simulink model "APA_AEB_Version_0_1"  (R2019a)
settings: Solver=FixedStepAuto  StartTime=0.0  StopTime=2  FixedStep=0.01  RelTol=1e-3
libraries: simulink x4, dspnetwork x1, autolibshared x1
(part 3 of 3)

== matlab function APA_AEB_Version_0_1/Resettable Single USS Tracking System/Single USS Tracking System ==
  settings: updateMethod=DISCRETE
  data: Obj_Single_USS_Lgtl input single; Track_Sigle_USS output single; Obj_Single_USS_Latl input single; Vehicle_Lgtl_Vel input single; Vehicle_Latl_Vel input single; Predict_time input single; State_Trans_F input single; State_Trans_P input single; Observation_H input single; DetectNoise_R input single; ProcessNoise_Q input single
function Track_Sigle_USS = Single_USS_Tracking_System(Obj_Single_USS_Lgtl,Obj_Single_USS_Latl,Vehicle_Lgtl_Vel,Vehicle_Latl_Vel,Predict_time,State_Trans_F,State_Trans_P,Observation_H,DetectNoise_R,ProcessNoise_Q)

Delta_x = Vehicle_Lgtl_Vel * Predict_time;
Delta_y = Vehicle_Latl_Vel * Predict_time;
Detection = zeros(12,4);
State_Trans_P_Update = zeros(4,4);
Track_Sigle_USS = single(zeros(12,4));
persistent Track_Object

if isempty(Track_Object)
    Track_Object = zeros(12,4);
    for index = 1:12
        [datalgtl,Lgtl_position_index] = min(abs(Obj_Single_USS_Lgtl(:,index)));
        [datalatl,Latl_position_index] = min(abs(Obj_Single_USS_Latl(:,index)));
        if datalgtl~=0 && datalatl~=0
            %
            Track_Object(index,1) = Obj_Single_USS_Lgtl(Lgtl_position_index,index);
            Track_Object(index,2) = Obj_Single_USS_Latl(Latl_position_index,index);
            Track_Object(index,3) = -1*Vehicle_Lgtl_Vel;
            Track_Object(index,4) = -1*Vehicle_Latl_Vel;
        else
            Track_Object(index,1) = Obj_Single_USS_Lgtl(Lgtl_position_index,index);
            Track_Object(index,2) = Obj_Single_USS_Latl(Latl_position_index,index);
            Track_Object(index,3) = 0;
            Track_Object(index,4) = 0;
        end
    end
    return
end

for Track_id = 1:12
    
    [datalgtl,Lgtl_position_index] = min(abs(Obj_Single_USS_Lgtl(:,Track_id)));
    [datalatl,Latl_position_index] = min(abs(Obj_Single_USS_Latl(:,Track_id)));
    
    if datalgtl~=0 && datalatl~=0
        %
        Detection(Track_id,1) = Obj_Single_USS_Lgtl(Lgtl_position_index,Track_id);
        Detection(Track_id,2) = Obj_Single_USS_Latl(Latl_position_index,Track_id);
        Detection(Track_id,3) = -1*Vehicle_Lgtl_Vel;
        Detection(Track_id,4) = -1*Vehicle_Latl_Vel;
    else
        Detection(Track_id,1) = Obj_Single_USS_Lgtl(Lgtl_position_index,Track_id);
        Detection(Track_id,2) = Obj_Single_USS_Latl(Latl_position_index,Track_id);
        Detection(Track_id,3) = 0;
        Detection(Track_id,4) = 0;
    end
    
    Track_Object_state = (Track_Object(Track_id,:))';
    Track_Object_state_Pred = State_Trans_F * Track_Object_state;
    State_Trans_P = State_Trans_F*State_Trans_P*State_Trans_F'+ProcessNoise_Q;
    Detection_t = Detection(Track_id,:);
    M_dist = sqrt((Track_Object_state_Pred(1,1)-Detection_t(1,1))^2 + (Track_Object_state_Pred(2,1)-Detection_t(1,2))^2);
    if M_dist < 2000
        %       
        Detection_pred = Observation_H*Track_Object_state_Pred;
        Innovation_S = Observation_H*State_Trans_P*Observation_H'+DetectNoise_R;
        KalmanGain_K = State_Trans_P*Observation_H'/Innovation_S;
        Track_Object_state_Update = Track_Object_state_Pred+KalmanGain_K*(Detection(Track_id,:)'-Detection_pred);
        State_Trans_P_Update = (eye(4,4)-KalmanGain_K*Observation_H)*State_Trans_P;
        Track_Object(Track_id,:) = Track_Object_state_Update;
    else
        Track_Object(Track_id,:) = Track_Object(Track_id,:);
    end
end
Track_Sigle_USS = single(Track_Object);
end

== matlab function APA_AEB_Version_0_1/Vehicle_Movement_Calculation ==
  data: Longitual_Velocity input single; Vehicle_Corner output single; Lateral_Velocity input single; Vehicle_predict_time input single; Brake_dist input single; Wheel_Angle input single; Axle_Length input single; Wheel_Base input single; Frt_Bump_dist input single; Rear_Bump_dist input single; Side_wheel_dist input single; CG_Offset_dist input single; Vehicle_Corner_t output single
function [Vehicle_Corner,Vehicle_Corner_t] = Vehicle_Movement_Calculation(Longitual_Velocity,Lateral_Velocity,Vehicle_predict_time,Brake_dist,Wheel_Angle,...
    Axle_Length,Wheel_Base,Frt_Bump_dist,Rear_Bump_dist,Side_wheel_dist,CG_Offset_dist)

Vehicle_Movement_Longitual = Longitual_Velocity*Vehicle_predict_time;
Vehicle_Movement_Lateral = Lateral_Velocity*Vehicle_predict_time;
Vehivle_Lgtl_Brake_dist = Brake_dist;
Vehivle_Latl_Brake_dist = Brake_dist*sin(Wheel_Angle);

Vehicle_Movement_Longitual = Vehicle_Movement_Longitual + Vehivle_Lgtl_Brake_dist;
Vehicle_Movement_Lateral = Vehicle_Movement_Lateral + Vehivle_Latl_Brake_dist;

Corner_LR_X = -1*Rear_Bump_dist;
Corner_LR_Y = -0.5*Wheel_Base;
Corner_RR_X = Corner_LR_X;
Corner_RR_Y = 0.5*Wheel_Base;
Corner_LF_X = Axle_Length + Frt_Bump_dist;
Corner_LF_Y = -0.5*Wheel_Base;
Corner_RF_X = Axle_Length + Frt_Bump_dist;
Corner_RF_Y = 0.5*Wheel_Base;

Corner_LR_X_t = -1*Rear_Bump_dist + Vehicle_Movement_Longitual;
Corner_LR_Y_t = -0.5*Wheel_Base + Vehicle_Movement_Lateral;
Corner_RR_X_t = Corner_LR_X + Vehicle_Movement_Longitual;
Corner_RR_Y_t = 0.5*Wheel_Base + Vehicle_Movement_Lateral;
Corner_LF_X_t = Axle_Length + Frt_Bump_dist + Vehicle_Movement_Longitual;
Corner_LF_Y_t = -0.5*Wheel_Base + Vehicle_Movement_Lateral;
Corner_RF_X_t = Axle_Length + Frt_Bump_dist + Vehicle_Movement_Longitual;
Corner_RF_Y_t = 0.5*Wheel_Base + Vehicle_Movement_Lateral;


Vehicle_Corner_Lgtl = [Corner_LR_X Corner_RR_X Corner_LF_X Corner_RF_X];
Vehicle_Corner_Latl = [Corner_LR_Y Corner_RR_Y Corner_LF_Y Corner_RF_Y];
Vehicle_Corner_Lgtl_t = [Corner_LR_X_t Corner_RR_X_t Corner_LF_X_t Corner_RF_X_t];
Vehicle_Corner_Latl_t = [Corner_LR_Y_t Corner_RR_Y_t Corner_LF_Y_t Corner_RF_Y_t];

Vehicle_Corner = [Vehicle_Corner_Lgtl;Vehicle_Corner_Latl];
Vehicle_Corner_t = [Vehicle_Corner_Lgtl_t;Vehicle_Corner_Latl_t];

== matlab function APA_AEB_Version_0_1/Collision Assessment/Switch Case Action Subsystem/Single_USS_Collision_Assessment ==
  data: Vehicle_Corner input single; Brake_Req_Flag output single; Vehicle_Corner_t input single; Obj_Single_USS_Lgtl input single; Obj_Single_USS_Latl input single

function Brake_Req_Flag = Single_USS_Collision_Assessment(Vehicle_Corner,Vehicle_Corner_t,Obj_Single_USS_Lgtl,Obj_Single_USS_Latl)
% coder.extrinsic('convhull')
%将输入的车辆坐标拆分
Vehicle_Corner_Lgtl = Vehicle_Corner ( 1 , : )'*100 ;
Vehicle_Corner_Latl = Vehicle_Corner ( 2 , : )' *100;
Vehicle_Corner_Lgtl_t = Vehicle_Corner_t( 1 , : )'*100 ;
Vehicle_Corner_Latl_t = Vehicle_Corner_t( 2 , : )'*100 ;
x_outline=[Vehicle_Corner_Lgtl ; Vehicle_Corner_Lgtl_t];
y_outline = [ Vehicle_Corner_Latl ; Vehicle_Corner_Latl_t ];

x_Obj_Single_USS = zeros(60,1);
y_Obj_Single_USS = zeros(60,1);
for k=1:1:12
    for i=1:1:5
    x_Obj_Single_USS((k-1)*5+i) = Obj_Single_USS_Lgtl(i,k);
    y_Obj_Single_USS((k-1)*5+i) = Obj_Single_USS_Latl(i,k);
    end
end
for i=1:1:60
    if x_Obj_Single_USS(i)==0&&y_Obj_Single_USS(i)==0
        x_Obj_Single_USS(i) = +inf ;
        y_Obj_Single_USS(i) = +inf ; 
    end
end
% %判断目标位置是否在车辆轮轮廓以内
[obstacle_in_trajector ] = inpolygon( x_Obj_Single_USS'*0.1 , y_Obj_Single_USS'*0.1 , x_outline , y_outline );
% [obstacle_in_trajector ] = inpolygon( Obj_Single_USS_Lgtl.*0.1 , Obj_Single_USS_Latl.*0.1 , x_outline' , y_outline' );
%是否刹车，若有目标点在轮廓内则发0刹车，反之发1不刹
if sum( obstacle_in_trajector )>0
Brake_Req_Flag = single(0);
else
Brake_Req_Flag = single(1);
end
% function Brake_Req_Flag = Single_USS_Collision_Assessment(Vehicle_Corner,Vehicle_Corner_t,Obj_Single_USS_Lgtl,Obj_Single_USS_Latl)
% %将输入的车辆坐标拆分
% Vehicle_Corner_Lgtl = Vehicle_Corner ( 1 , : )' ;
% Vehicle_Corner_Latl = Vehicle_Corner ( 2 , : )' ;
% Vehicle_Corner_Lgtl_t = Vehicle_Corner_t( 1 , : )' ;
% Vehicle_Corner_Latl_t = Vehicle_Corner_t( 1 , : )' ;
% %找到预测后车辆角点在这一时刻车辆位姿内的角点
% [Vehicle_Corner_t_in_Vehicle_Corner ] = inpolygon( Vehicle_Corner_Lgtl_t , Vehicle_Corner_Latl_t , Vehicle_Corner_Lgtl , Vehicle_Corner_Latl );
% Vehicle_Corner_t_out_Vehicle_Corner_index = find( ~Vehicle_Corner_t_in_Vehicle_Corner );
% %找到这一时刻车辆角点在预测后车辆位姿内的角点在
% [Vehicle_Corner_in_Vehicle_Corner_t ] = inpolygon( Vehicle_Corner_Lgtl , Vehicle_Corner_Latl  , Vehicle_Corner_Lgtl_t , Vehicle_Corner_Latl_t );
% Vehicle_Corner_out_Vehicle_Corner_t_index = find( ~Vehicle_Corner_in_Vehicle_Corner_t );
% %写这一时刻和预测后车辆位姿的外轮廓矩阵
% Vehicle_Corner_t_out_num = length(Vehicle_Corner_t_out_Vehicle_Corner_index) ; 
% Vehicle_Corner_out_num =  length(Vehicle_Corner_out_Vehicle_Corner_t_index)   ; 
% outline_num = Vehicle_Corner_t_out_num + Vehicle_Corner_out_num ;                %轮廓的总点数
% x_outline = zeros(1,outline_num) ; 
% y_outline = zeros(1,outline_num) ; 
% for i=1:1:outline_num 
%     if i<= Vehicle_Corner_t_out_num
%     x_outline(i) = Vehicle_Corner_Lgtl_t( Vehicle_Corner_t_out_Vehicle_Corner_index(i) ) ; 
%     y_outline(i) = Vehicle_Corner_Latl_t( Vehicle_Corner_t_out_Vehicle_Corner_index(i) ) ;
%     else
%     x_outline(i) = Vehicle_Corner_Lgtl( Vehicle_Corner_out_Vehicle_Corner_t_index(i-Vehicle_Corner_t_out_num) ) ; 
%     y_outline(i) = Vehicle_Corner_Latl( Vehicle_Corner_out_Vehicle_Corner_t_index(i-Vehicle_Corner_t_out_num) ) ;
%     end
% end
% %判断目标位置是否在车辆轮轮廓以内
% [obstacle_in_trajector ] = inpolygon( Obj_Single_USS_Lgtl , Obj_Single_USS_Latl , x_outline' , y_outline' );
% %是否刹车，若有目标点在轮廓内则发0刹车，反之发1不刹
% if sum( obstacle_in_trajector )>0
% Brake_Req_Flag = 0;
% else
% Brake_Req_Flag = 1;
% end

== matlab function APA_AEB_Version_0_1/Collision Assessment/Switch Case Action Subsystem1/Multi_USS_Collision_Assessment ==
  data: Vehicle_Corner input single; Brake_Req_Flag output single; Vehicle_Corner_t input single; Obj_Triangle_USS_Lgtl input single; Obj_Triangle_USS_Latl input single

function Brake_Req_Flag = Multi_USS_Collision_Assessment(Vehicle_Corner,Vehicle_Corner_t,Obj_Triangle_USS_Lgtl,Obj_Triangle_USS_Latl)
% coder.extrinsic('convhull')
Vehicle_Corner_Lgtl = Vehicle_Corner ( 1 , : )'*100 ;
Vehicle_Corner_Latl = Vehicle_Corner ( 2 , : )' *100;
Vehicle_Corner_Lgtl_t = Vehicle_Corner_t( 1 , : )'*100 ;
Vehicle_Corner_Latl_t = Vehicle_Corner_t( 2 , : )'*100 ;
x_outline=[Vehicle_Corner_Lgtl ;Vehicle_Corner_Lgtl_t];
y_outline = [ Vehicle_Corner_Latl;Vehicle_Corner_Latl_t ];

%将0变为正无穷
for i=1:1:6
    if Obj_Triangle_USS_Lgtl(i)==0&&Obj_Triangle_USS_Latl(i)==0
        Obj_Triangle_USS_Lgtl(i) = +inf ;
        Obj_Triangle_USS_Latl(i) = +inf ; 
    end
end
%判断目标位置是否在车辆轮轮廓以内
[obstacle_in_trajector ] = inpolygon( Obj_Triangle_USS_Lgtl'*0.1 , Obj_Triangle_USS_Latl'*0.1 , x_outline , y_outline );
%是否刹车，若有目标点在轮廓内则发0刹车，反之发1不刹
if sum( obstacle_in_trajector )>0
Brake_Req_Flag = single(0);
else
Brake_Req_Flag = single(1);
end

== matlab function APA_AEB_Version_0_1/Ultarsonic Processment /Subsystem1/Subsystem1/Detection Processment/Switch Case Action Subsystem1/MATLAB Function ==
  data: Sensor_Detection input; Longitudial_triDist output; Lateral_triDist output
function [Longitudial_triDist,Lateral_triDist] = fcn(Sensor_Detection)
    %
    Longitudial_triDist = single(zeros(1,6));
    %
    Lateral_triDist = single(zeros(1,6));
    %
    Front_leftFront_uss_position_x  = single(3528.8);
    %
    Front_leftFront_uss_position_y  = single(-650.5);
    %
    Front_leftMiddle_uss_position_x  = single(3673.9);
    %
    Front_leftMiddle_uss_position_y  = single(-320.3);
    %
    Front_rightMiddle_uss_position_x  = single(3673.9);
    %
    Front_rightMiddle_uss_position_y  = single(320.3);
    %
    Front_rightFront_uss_position_x  =  single(3528.7);
    %
    Front_rightFront_uss_position_y  =  single(650.4);
    %
    Rear_leftRear_uss_position_x  =  single(-784.2);
    %
    Rear_leftRear_uss_position_y  =  single(-660.4);
    %
    Rear_leftMiddle_uss_position_x  =  single(-904.5);
    %
    Rear_leftMiddle_uss_position_y  =  single(-280.4);
    %
    Rear_rightMiddle_uss_position_x  =  single(-904.5);
    %
    Rear_rightMiddle_uss_position_y  =  single(280.4);
    %
    Rear_rightRear_uss_position_x  =  single(-784.2);
    %
    Rear_rightRear_uss_position_y  =  single(660.4);
    %
    USS_dist  = [single(sqrt((Front_leftFront_uss_position_x-Front_leftMiddle_uss_position_x)^2+(Front_leftFront_uss_position_y-Front_leftMiddle_uss_position_y)^2)),...
        single(sqrt((Front_rightMiddle_uss_position_x-Front_leftMiddle_uss_position_x)^2+(Front_rightMiddle_uss_position_y-Front_leftMiddle_uss_position_y)^2)),...
        single(sqrt((Front_rightMiddle_uss_position_x-Front_rightFront_uss_position_x)^2+(Front_rightMiddle_uss_position_y-Front_rightFront_uss_position_x)^2)),...
        single(sqrt((Rear_rightMiddle_uss_position_x-Rear_rightRear_uss_position_x)^2+(Rear_rightMiddle_uss_position_y-Rear_rightRear_uss_position_y)^2)),...
        single(sqrt((Rear_rightMiddle_uss_position_x-Rear_leftMiddle_uss_position_x)^2+(Rear_rightMiddle_uss_position_y-Rear_leftMiddle_uss_position_y)^2)),...
        single(sqrt((Rear_leftRear_uss_position_x-Rear_leftMiddle_uss_position_x)^2+(Rear_leftRear_uss_position_y-Rear_leftMiddle_uss_position_y)^2))];

    
    
    if Sensor_Detection(2)>0 && Sensor_Detection(3)>0 && Sensor_Detection(4)==0 && Sensor_Detection(2)+Sensor_Detection(3) > USS_dist(1)
        alpha = single(acos((USS_dist(1)^2+Sensor_Detection(2)^2-Sensor_Detection(3)^2)/(2 * USS_dist(1) * Sensor_Detection(2))));
        x = single(sin(alpha)*Sensor_Detection(2));
        y = single(cos(alpha)*Sensor_Detection(2)); 
        a = (Front_leftMiddle_uss_position_x - Front_leftFront_uss_position_x)/USS_dist(1);
        b= abs(Front_leftMiddle_uss_position_y - Front_leftFront_uss_position_y)/USS_dist(1);
        Longitudial_triDist(1) = x * b + y * a + Front_leftFront_uss_position_x;
        Lateral_triDist(1) = - x * a + y * b + Front_leftFront_uss_position_y;
    end
    
    if Sensor_Detection(3)>0 && Sensor_Detection(4)>0 && Sensor_Detection(2)==0 && Sensor_Detection(5)==0 && Sensor_Detection(3)+Sensor_Detection(4) > USS_dist(2)
            alpha = acos((USS_dist(2)^2+Sensor_Detection(3)^2-Sensor_Detection(4)^2)/(2 * USS_dist(2) * Sensor_Detection(3)));
            x = sin(alpha)*Sensor_Detection(3);
            y = cos(alpha)*Sensor_Detection(3);
            a = (Front_rightMiddle_uss_position_x - Front_leftMiddle_uss_position_x)/USS_dist(2);
            b = abs(Front_rightMiddle_uss_position_y - Front_leftMiddle_uss_position_y)/USS_dist(2);
            Longitudial_triDist(2) = x * b + y * a + Front_leftMiddle_uss_position_x;
            Lateral_triDist(2) = - x * a + y * b + Front_leftMiddle_uss_position_y;
    end
    
    if Sensor_Detection(4)>0 && Sensor_Detection(5)>0 && Sensor_Detection(3)==0 && Sensor_Detection(4)+Sensor_Detection(5) > USS_dist(3)
        alpha = acos((USS_dist(3)^2+Sensor_Detection(4)^2-Sensor_Detection(5)^2)/(2 * USS_dist(3) * Sensor_Detection(4)));
        x = sin(alpha)*Sensor_Detection(4);
        y = cos(alpha)*Sensor_Detection(4);
        a = (Front_rightFront_uss_position_x - Front_rightMiddle_uss_position_x)/USS_dist(3);
        b = abs(Front_rightFront_uss_position_y - Front_rightMiddle_uss_position_y)/USS_dist(3);
        Longitudial_triDist(3) = x * b + y * a + Front_rightMiddle_uss_position_x;
        Lateral_triDist(3) = - x * a + y * b + Front_rightMiddle_uss_position_y;
    end
    
    if Sensor_Detection(8)>0 && Sensor_Detection(9)>0 && Sensor_Detection(10)==0 && Sensor_Detection(8)+Sensor_Detection(9) > USS_dist(4)
        alpha = acos((USS_dist(4)^2+Sensor_Detection(8)^2-Sensor_Detection(9)^2)/(2 * USS_dist(4) * Sensor_Detection(8)));
        x = sin(alpha) * Sensor_Detection(8);
        y = cos(alpha )* Sensor_Detection(8); 
        a = -(Rear_rightMiddle_uss_position_x - Rear_rightRear_uss_position_x)/USS_dist(4);
        b= abs(Rear_rightMiddle_uss_position_y - Rear_rightRear_uss_position_y)/USS_dist(4);
        Longitudial_triDist(4) = - ( x * b + y * a ) + Rear_rightRear_uss_position_x;
        Lateral_triDist(4) = - ( - x * a + y * b ) + Rear_rightRear_uss_position_y;
    end
    
    if Sensor_Detection(9)>0 && Sensor_Detection(10)>0 && Sensor_Detection(8)==0 && Sensor_Detection(11)==0 && Sensor_Detection(9)+Sensor_Detection(10) > USS_dist(5)
        alpha = acos((USS_dist(5)^2+Sensor_Detection(9)^2-Sensor_Detection(10)^2)/(2 * USS_dist(5) * Sensor_Detection(9)));
        x = sin(alpha)*Sensor_Detection(9);
        y = cos(alpha)*Sensor_Detection(9); 
        a = -(Rear_leftMiddle_uss_position_x - Rear_rightMiddle_uss_position_x)/USS_dist(5);
        b= abs(Rear_leftMiddle_uss_position_y - Rear_rightMiddle_uss_position_y)/USS_dist(5);
        Longitudial_triDist(5) = - ( x * b + y * a ) + Rear_rightMiddle_uss_position_x;
        Lateral_triDist(5) = - ( x * a + y * b ) + Rear_rightMiddle_uss_position_y;
    end
    
    if Sensor_Detection(10)>0 && Sensor_Detection(11)>0 && Sensor_Detection(9)==0 && Sensor_Detection(10)+Sensor_Detection(11) > USS_dist(6)
        alpha = acos((USS_dist(6)^2+Sensor_Detection(10)^2-Sensor_Detection(11)^2)/(2 * USS_dist(6) * Sensor_Detection(10)));
        x = sin(alpha)*Sensor_Detection(10);
        y = cos(alpha)*Sensor_Detection(10); 
        a = -(Rear_leftRear_uss_position_x - Rear_leftMiddle_uss_position_x)/USS_dist(6);
        b= abs(Rear_leftRear_uss_position_y - Rear_leftMiddle_uss_position_y)/USS_dist(6);
        Longitudial_triDist(6) = - ( x * b + y * a ) + Rear_leftMiddle_uss_position_x;
        Lateral_triDist(6) = - ( - x * a + y * b ) + Rear_leftMiddle_uss_position_y;
    end

== matlab function APA_AEB_Version_0_1/Multi_USS_Tracking_System/Multi USS Tracking ==
  settings: updateMethod=DISCRETE
  data: Obj_Triangle_USS_Lgtl input single; Track_Multi_USS output single; Obj_Triangle_USS_Latl input single; Vehicle_Lgtl_Vel input single; Vehicle_Latl_Vel input single; Predict_time input single; State_Trans_F input single; State_Trans_P input single; Observation_H input single; DetectNoise_R input single; ProcessNoise_Q input single
function Track_Multi_USS = Multi_USS_Tracking_System(Obj_Triangle_USS_Lgtl,Obj_Triangle_USS_Latl,Vehicle_Lgtl_Vel,Vehicle_Latl_Vel,Predict_time,State_Trans_F,State_Trans_P,Observation_H,DetectNoise_R,ProcessNoise_Q)

Delta_x_M = Vehicle_Lgtl_Vel * Predict_time;
Delta_y_M = Vehicle_Latl_Vel * Predict_time;
Detection_M = zeros(6,4);
State_Trans_P_Update_M = zeros(4,4);
Track_Multi_USS = single(zeros(6,4));

persistent Track_Object_Multi

if isempty(Track_Object_Multi)
    % Init the global params for tracker
    Track_Object_Multi = zeros(6,4);
    
    for index_M = 1:6
        if Obj_Triangle_USS_Lgtl(index_M)~=0 && Obj_Triangle_USS_Latl(index_M)~=0
            %
            Track_Object_Multi(index_M,1) = Obj_Triangle_USS_Lgtl(index_M);
            Track_Object_Multi(index_M,2) = Obj_Triangle_USS_Latl(index_M);
            Track_Object_Multi(index_M,3) = -1*Vehicle_Lgtl_Vel;
            Track_Object_Multi(index_M,4) = -1*Vehicle_Latl_Vel;
        else
            Track_Object_Multi(index_M,1) = Obj_Triangle_USS_Lgtl(index_M);
            Track_Object_Multi(index_M,2) = Obj_Triangle_USS_Latl(index_M);
            Track_Object_Multi(index_M,3) = 0;
            Track_Object_Multi(index_M,4) = 0;
        end
    end
    return;
end

for Track_id_M = 1:6
    %
    if Obj_Triangle_USS_Lgtl(Track_id_M)~=0 && Obj_Triangle_USS_Latl(Track_id_M)~=0
        Detection_M(Track_id_M,1) = Obj_Triangle_USS_Lgtl(Track_id_M);
        Detection_M(Track_id_M,2) = Obj_Triangle_USS_Latl(Track_id_M);
        Detection_M(Track_id_M,3) = -1*Vehicle_Lgtl_Vel;
        Detection_M(Track_id_M,4) = -1*Vehicle_Latl_Vel;
    else
        Detection_M(Track_id_M,1) = Obj_Triangle_USS_Lgtl(Track_id_M);
        Detection_M(Track_id_M,2) = Obj_Triangle_USS_Latl(Track_id_M);
        Detection_M(Track_id_M,3) = 0;
        Detection_M(Track_id_M,4) = 0;
    end
    %Kalman——Filter
    Track_Object_state_M = (Track_Object_Multi(Track_id_M,:))';
    Track_Object_state_Pred_M = State_Trans_F * Track_Object_state_M;
    State_Trans_P = State_Trans_F*State_Trans_P*State_Trans_F'+ProcessNoise_Q;
    Detection_M_t = Detection_M(Track_id_M,:);
    MM_dist = sqrt((Track_Object_state_Pred_M(1,1)-Detection_M_t(1,1))^2 + (Track_Object_state_Pred_M(2,1)-Detection_M_t(1,2))^2);
    if MM_dist < 50000
        %
        Detection_pred_M = Observation_H*Track_Object_state_Pred_M;
        Innovation_S = Observation_H*State_Trans_P*Observation_H'+DetectNoise_R;
        KalmanGain_K = State_Trans_P*Observation_H'/Innovation_S;
        Track_Object_state_Update_M = Track_Object_state_Pred_M+KalmanGain_K*(Detection_M(Track_id_M,:)'-Detection_pred_M);
        State_Trans_P_Update = (eye(4,4)-KalmanGain_K*Observation_H)*State_Trans_P;    
        Track_Object_Multi(Track_id_M,:) = Track_Object_state_Update_M;
    else
        Track_Object_Multi(Track_id_M,:) = Track_Object_Multi(Track_id_M,:);
    end
end
Track_Multi_USS = single(Track_Object_Multi);
end

== matlab function APA_AEB_Version_0_1/USS Wall HMI/USS_Wall_HMI ==
  data: single_Lgtl input single; output1 output single; single_Latl input single; triangle_Lgtl input single; triangle_Latl input single; output2 output single; output3 output single; output4 output single
% single_Lgtl,single_Latl:12个雷达探测到障碍物的x,y；triangle_Lgtl,triangle_Latl:6个三角定位区域内的x,y
% single_Lgtl:5*12 ；single_Latl:5*12 ；triangle_Lgtl:1*6 ；triangle_Latl:1*6
% 车宽取1.606，坐标原点在车后轴中心上
% ux:1*4 ；sy:1*4
function [output1, output2, output3, output4] = USS_Wall_HMI(single_Lgtl, single_Latl, triangle_Lgtl, triangle_Latl)
%#codegen
vehicle_w = 1606;
Lgtl = zeros(1,4);
Latl = zeros(1,4);
%% 按y大小分成4个部分,记录sy,ty中位于4个部分的y坐标值在sy,ty矩阵中的位置，都是n行2列的矩阵
part1_singleLatl = []; part1_triangleLatl = [];
part2_singleLatl = []; part2_triangleLatl = [];
part3_singleLatl = []; part3_triangleLatl = [];
part4_singleLatl = []; part4_triangleLatl = [];
for singleLatl_row = 1:size(single_Latl,1)
    for singleLatl_col = 1:size(single_Latl,2)
        if single_Latl(singleLatl_row, singleLatl_col) < -(vehicle_w/4) && single_Latl(singleLatl_row, singleLatl_col) >= -vehicle_w/2
            part1_singleLatl = [part1_singleLatl; singleLatl_row, singleLatl_col];
        end
        if single_Latl(singleLatl_row, singleLatl_col) >= -(vehicle_w/4) && single_Latl(singleLatl_row, singleLatl_col) < 0
            part2_singleLatl = [part2_singleLatl; singleLatl_row, singleLatl_col];
        end
        if single_Latl(singleLatl_row, singleLatl_col) >= 0 && single_Latl(singleLatl_row, singleLatl_col) < vehicle_w/4
            part3_singleLatl = [part3_singleLatl; singleLatl_row, singleLatl_col];
        end
        if single_Latl(singleLatl_row, singleLatl_col) >= vehicle_w/4 && single_Latl(singleLatl_row, singleLatl_col) <= vehicle_w/2
            part4_singleLatl = [part4_singleLatl; singleLatl_row, singleLatl_col];
        end
    end
end
for triangleLatl_row = 1:size(triangle_Latl,1)
    for triangleLatl_col = 1:size(triangle_Latl,2)
        if triangle_Latl(triangleLatl_row, triangleLatl_col) < -(vehicle_w/4) && single_Latl(singleLatl_row, singleLatl_col) >= -vehicle_w/2
            part1_triangleLatl = [part1_triangleLatl; triangleLatl_row, triangleLatl_col];
        end
        if triangle_Latl(triangleLatl_row, triangleLatl_col) >= -(vehicle_w/4) && triangle_Latl(triangleLatl_row, triangleLatl_col) < 0
            part2_triangleLatl = [part2_triangleLatl; triangleLatl_row, triangleLatl_col];
        end
        if triangle_Latl(triangleLatl_row, triangleLatl_col) >= 0 && triangle_Latl(triangleLatl_row, triangleLatl_col) < vehicle_w/4
            part3_triangleLatl = [part3_triangleLatl; triangleLatl_row, triangleLatl_col];
        end
        if triangle_Latl(triangleLatl_row, triangleLatl_col) >= vehicle_w/4 && triangle_Latl(triangleLatl_row, triangleLatl_col) <= vehicle_w/2
            part4_triangleLatl = [part4_triangleLatl; triangleLatl_row, triangleLatl_col];
        end
    end
end
%% 找各个区域内x>0的最小值，并根据其在sx,tx中的位置找到对应的y值，输出给ux,uy
Lgtl(1) = max(max(max(single_Lgtl)),max(triangle_Lgtl)); 
if ~isempty(part1_singleLatl)
    for singleLgtl1_col = 1:size(part1_singleLatl,1)
        if single_Lgtl(part1_singleLatl(singleLgtl1_col,1), part1_singleLatl(singleLgtl1_col,2)) > 0 && single_Lgtl(part1_singleLatl(singleLgtl1_col,1), part1_singleLatl(singleLgtl1_col,2)) <= Lgtl(1)
            Lgtl(1) = single_Lgtl(part1_singleLatl(singleLgtl1_col,1), part1_singleLatl(singleLgtl1_col,2));
            Latl(1) = single_Latl(part1_singleLatl(singleLgtl1_col,1), part1_singleLatl(singleLgtl1_col,2));
        end
    end
end
if ~isempty(part1_triangleLatl)
    for triangleLgtl1_col = 1:size(part1_triangleLatl,1)
        if triangle_Lgtl(part1_triangleLatl(triangleLgtl1_col,1), part1_triangleLatl(triangleLgtl1_col,2)) > 0 && triangle_Lgtl(part1_triangleLatl(triangleLgtl1_col,1), part1_triangleLatl(triangleLgtl1_col,2)) <= Lgtl(1)
            Lgtl(1) = triangle_Lgtl(part1_triangleLatl(triangleLgtl1_col,1), part1_triangleLatl(triangleLgtl1_col,2));
            Latl(1) = triangle_Latl(part1_triangleLatl(triangleLgtl1_col,1), part1_triangleLatl(triangleLgtl1_col,2));
        end
    end
end

Lgtl(2) = max(max(max(single_Lgtl)),max(triangle_Lgtl));
if ~isempty(part2_singleLatl)
    for singleLgtl2_col = 1:size(part2_singleLatl,1)
        if single_Lgtl(part2_singleLatl(singleLgtl2_col,1), part2_singleLatl(singleLgtl2_col,2)) > 0 && single_Lgtl(part2_singleLatl(singleLgtl2_col,1), part2_singleLatl(singleLgtl2_col,2)) <= Lgtl(2)
            Lgtl(2) = single_Lgtl(part2_singleLatl(singleLgtl2_col,1), part2_singleLatl(singleLgtl2_col,2));
            Latl(2) = single_Latl(part2_singleLatl(singleLgtl2_col,1), part2_singleLatl(singleLgtl2_col,2));
        end
    end
end
if ~isempty(part2_triangleLatl)
    for triangleLgtl2_col = 1:size(part2_triangleLatl,1)
        if triangle_Lgtl(part2_triangleLatl(triangleLgtl2_col,1), part2_triangleLatl(triangleLgtl2_col,2)) > 0 && triangle_Lgtl(part2_triangleLatl(triangleLgtl2_col,1), part2_triangleLatl(triangleLgtl2_col,2)) <= Lgtl(2)
            Lgtl(2) = triangle_Lgtl(part2_triangleLatl(triangleLgtl2_col,1), part2_triangleLatl(triangleLgtl2_col,2));
            Latl(2) = triangle_Latl(part2_triangleLatl(triangleLgtl2_col,1), part2_triangleLatl(triangleLgtl2_col,2));
        end
    end
end

Lgtl(3) = max(max(max(single_Lgtl)),max(triangle_Lgtl));
if ~isempty(part3_singleLatl)
    for singleLgtl3_col = 1:size(part3_singleLatl,1)
        if single_Lgtl(part3_singleLatl(singleLgtl3_col,1), part3_singleLatl(singleLgtl3_col,2)) > 0 && single_Lgtl(part3_singleLatl(singleLgtl3_col,1), part3_singleLatl(singleLgtl3_col,2)) <= Lgtl(3)
            Lgtl(3) = single_Lgtl(part3_singleLatl(singleLgtl3_col,1), part3_singleLatl(singleLgtl3_col,2));
            Latl(3) = single_Latl(part3_singleLatl(singleLgtl3_col,1), part3_singleLatl(singleLgtl3_col,2));
        end
    end
end
if ~isempty(part3_triangleLatl)
    for triangleLgtl3_col = 1:size(part3_triangleLatl,1)
        if triangle_Lgtl(part3_triangleLatl(triangleLgtl3_col,1), part3_triangleLatl(triangleLgtl3_col,2)) > 0 && triangle_Lgtl(part3_triangleLatl(triangleLgtl3_col,1), part3_triangleLatl(triangleLgtl3_col,2)) <= Lgtl(3)
            Lgtl(3) = triangle_Lgtl(part3_triangleLatl(triangleLgtl3_col,1), part3_triangleLatl(triangleLgtl3_col,2));
            Latl(3) = triangle_Latl(part3_triangleLatl(triangleLgtl3_col,1), part3_triangleLatl(triangleLgtl3_col,2));
        end
    end
end

Lgtl(4) = max(max(max(single_Lgtl)),max(triangle_Lgtl));
if ~isempty(part4_singleLatl)
    for singleLgtl4_col = 1:size(part4_singleLatl,1)
        if single_Lgtl(part4_singleLatl(singleLgtl4_col,1), part4_singleLatl(singleLgtl4_col,2)) > 0 && single_Lgtl(part4_singleLatl(singleLgtl4_col,1), part4_singleLatl(singleLgtl4_col,2)) <= Lgtl(4)
            Lgtl(4) = single_Lgtl(part4_singleLatl(singleLgtl4_col,1), part4_singleLatl(singleLgtl4_col,2));
            Latl(4) = single_Latl(part4_singleLatl(singleLgtl4_col,1), part4_singleLatl(singleLgtl4_col,2));
        end
    end
end
if ~isempty(part4_triangleLatl)
    for triangleLgtl4_col = 1:size(part4_triangleLatl,1)
        if triangle_Lgtl(part4_triangleLatl(triangleLgtl4_col,1), part4_triangleLatl(triangleLgtl4_col,2)) > 0 && triangle_Lgtl(part4_triangleLatl(triangleLgtl4_col,1), part4_triangleLatl(triangleLgtl4_col,2)) <= Lgtl(4)
            Lgtl(4) = triangle_Lgtl(part4_triangleLatl(triangleLgtl4_col,1), part4_triangleLatl(triangleLgtl4_col,2));
            Latl(4) = triangle_Latl(part4_triangleLatl(triangleLgtl4_col,1), part4_triangleLatl(triangleLgtl4_col,2));
        end
    end
end
%% output[x,y,d,flag]
for Latl_col = 1:size(Latl,2)
    if Latl(Latl_col) == 0
        Lgtl(Latl_col) = 0;
    end
end
output1=zeros(1,4);
output2=zeros(1,4);
output3=zeros(1,4);
output4=zeros(1,4);
if Lgtl(1) ~= 0
    output1(1) = Lgtl(1);
    output1(2) = Latl(1);
    output1(3) = sqrt(Lgtl(1)^2+Latl(1)^2);
    output1(4) = 1;
end
if Lgtl(2) ~= 0
    output2(1) = Lgtl(2);
    output2(2) = Latl(2);
    output2(3) = sqrt(Lgtl(2)^2+Latl(2)^2);
    output2(4) = 1;
end
if Lgtl(3) ~= 0
    output3(1) = Lgtl(3);
    output3(2) = Latl(3);
    output3(3) = sqrt(Lgtl(3)^2+Latl(3)^2);
    output3(4) = 1;
end
if Lgtl(4) ~= 0
    output4(1) = Lgtl(4);
    output4(2) = Latl(4);
    output4(3) = sqrt(Lgtl(4)^2+Latl(4)^2);
    output4(4) = 1;
end

== matlab function APA_AEB_Version_0_1/Track Management & Reset ==
  data: Track_Sigle_USS input single; Global_Tracker_AEB output single; Track_Multi_USS input single; Obj_Single_USS_Lgtl input single; Obj_Single_USS_Latl input single; Obj_Triangle_USS_Lgtl input single; Obj_Triangle_USS_Latl input single; Brake_Req_single input single; Brake_Req_Multi input single; Reset_Flag_S output single; Reset_Flag_M output single; c output single
function [Global_Tracker_AEB,...
    Reset_Flag_S,...
    Reset_Flag_M,c] = Track_Management(Track_Sigle_USS,Track_Multi_USS,Obj_Single_USS_Lgtl,Obj_Single_USS_Latl,Obj_Triangle_USS_Lgtl,Obj_Triangle_USS_Latl,Brake_Req_single,Brake_Req_Multi)

persistent Global_Tracker Sgl_USS_Reset_Flag Multi_USS_Reset_Flag Countyy

if isempty(Global_Tracker) && isempty(Sgl_USS_Reset_Flag) && isempty(Multi_USS_Reset_Flag)
    %
    Global_Tracker = [Track_Sigle_USS;Track_Multi_USS];  
    Sgl_USS_Reset_Flag = 0;
    Multi_USS_Reset_Flag = 0;
    Countyy = 0;
end

if (Brake_Req_single || Brake_Req_Multi) == 0 
    
    %没有制动触发，局部的跟踪器传值
    Global_Tracker = [Track_Sigle_USS;Track_Multi_USS];
    
    Sgl_USS_Reset_Flag = 0;
    
    Multi_USS_Reset_Flag = 0;
else
    %有制动触发
    Dist = zeros(18,1);
    for i = 1:12
        [datalgtl,Lgtl_position_index] = min(abs(Obj_Single_USS_Lgtl(:,i)));
        [datalatl,Latl_position_index] = min(abs(Obj_Single_USS_Latl(:,i)));
        Dist(i,1) = sqrt((Global_Tracker(i,1)-datalgtl)^2 + (Global_Tracker(i,2)-datalatl)^2);
        if Dist(i,1)<50
            Global_Tracker(i,:) = Track_Sigle_USS(i,:);
            Sgl_USS_Reset_Flag = 1;
%             Countyy = Countyy +1;
        else
            Countyy = Countyy +1;
        end
    end
    for j = 1:6
        [datalgtl,Lgtl_position_index] = min(abs(Obj_Triangle_USS_Lgtl(:,j)));
        [datalatl,Latl_position_index] = min(abs(Obj_Triangle_USS_Latl(:,j)));
        Dist(j+12,1) = sqrt((Global_Tracker(j+6,1)-datalgtl)^2 + (Global_Tracker(j+6,2)-datalatl)^2);
        if Dist(i,1)<50
            Global_Tracker(j+12,:) = Track_Multi_USS(j,:);
            Multi_USS_Reset_Flag = 1;
%             Countyy = Countyy +1;
        else
            Countyy = Countyy +1;
        end
    end
    if Countyy == 50
        Sgl_USS_Reset_Flag = 1;
        Multi_USS_Reset_Flag = 1;
    elseif Countyy == 52
        Sgl_USS_Reset_Flag = 0;
        Multi_USS_Reset_Flag = 0;
        Countyy =0;
    end
end

% disp(Countyy)
Global_Tracker_AEB = Global_Tracker;
Reset_Flag_S = single(Sgl_USS_Reset_Flag);
Reset_Flag_M = single(Multi_USS_Reset_Flag);
c = single(Countyy);
